simulink model "IB_BIEN_y_TG_BIEN"  (Simulink 8.1)
settings: Solver=ode45  StartTime=0.0  StopTime=50  RelTol=1e-3
PreLoadFcn:
  | Initial_datab
  | Const_IB
values from neighbouring files (symbols this model uses):
  a1 = (Iyy-Izz)/Ixx    (= -1.125)    [Initial_datab.m]
  a2 = Jr/Ixx    (= 0.00697115384615)    [Initial_datab.m]
  a3 = (Izz-Ixx)/Iyy    (= 1.11607142857)    [Initial_datab.m]
  a5 = (Ixx-Iyy)/Izz    (= -0.0349344978166)    [Initial_datab.m]
  alp1 = 20    [Initial_datab.m]
  alp2 = 10    [Initial_datab.m]
  b = 1.2*10^(-4)    (= 0.00012)    [Initial_datab.m]
  b1 = 1/Ixx    (= 96.1538461538)    [Initial_datab.m]
  b2 = 1/Iyy    (= 89.2857142857)    [Initial_datab.m]
  b3 = 1/Izz    (= 43.6681222707)    [Initial_datab.m]
  c1 = 10    [Const_IB.m]
  c10 = 0.75    [Const_IB.m]
  c11 = 1    [Const_IB.m]
  c12 = 0.75    [Const_IB.m]
  c2 = 6    [Const_IB.m]
  c3 = 10    [Const_IB.m]
  c4 = 6    [Const_IB.m]
  c5 = 2    [Const_IB.m]
  c6 = 2    [Const_IB.m]
  c7 = 3.5    [Const_IB.m]
  c8 = 1.5    [Const_IB.m]
  c9 = 1    [Const_IB.m]
  d = 3*10^(-6)    (= 3e-06)    [Initial_datab.m]
  Ixx = 10.4*10^(-3)    (= 0.0104)    [Initial_datab.m]
  Iyy = 11.2*10^(-3)    (= 0.0112)    [Initial_datab.m]
  Izz = 2.29*10^(-2)    (= 0.0229)    [Initial_datab.m]
  Jr = 7.25*10^(-5)    (= 7.25e-05)    [Initial_datab.m]
  k1x = -k1x    (= -0.5)    [Initial_datab.m]
  k1y = -k1y    (= -0.5)    [Initial_datab.m]
  k1z = -k1z    (= -2)    [Initial_datab.m]
  l = 0.225    [Initial_datab.m]
  ld1 = 0.07    [Const_IB.m]
  ld2 = 0.05    [Const_IB.m]
  ld3 = 0.01    [Const_IB.m]
  ld4 = 0.01    [Const_IB.m]
  ld5 = 0.001    [Const_IB.m]
  ld6 = 0.001    [Const_IB.m]
  m = 1.14    [Initial_datab.m]
  phi0 = 0    [Initial_datab.m]
  phi0dot = 0    [Initial_datab.m]
  psi0 = 0    [Initial_datab.m]
  psi0dot = 0    [Initial_datab.m]
  theta0 = 0    [Initial_datab.m]
  theta0dot = 0    [Initial_datab.m]
  x0 = 0    [Initial_datab.m]
  x0dot = 0    [Initial_datab.m]
  xf = -5    [Initial_datab.m]
  xfdot = 0    [Initial_datab.m]
  y0 = 0    [Initial_datab.m]
  y0dot = 0    [Initial_datab.m]
  yf = 5    [Initial_datab.m]
  yfdot = 0    [Initial_datab.m]
  z0 = 0    [Initial_datab.m]
  z0dot = 0    [Initial_datab.m]
  zf = 50    [Initial_datab.m]
  zfdot = 0    [Initial_datab.m]
undefined symbols (not defined in the file or in its folder): sigbuilder_block
(part 1 of 2)
settings Model: Creator=Ana  LastModifiedBy=Admin
settings SolverCC: MaxConsecutiveMinStep=5
settings DebuggingCC: StrictBusMsg=Warning

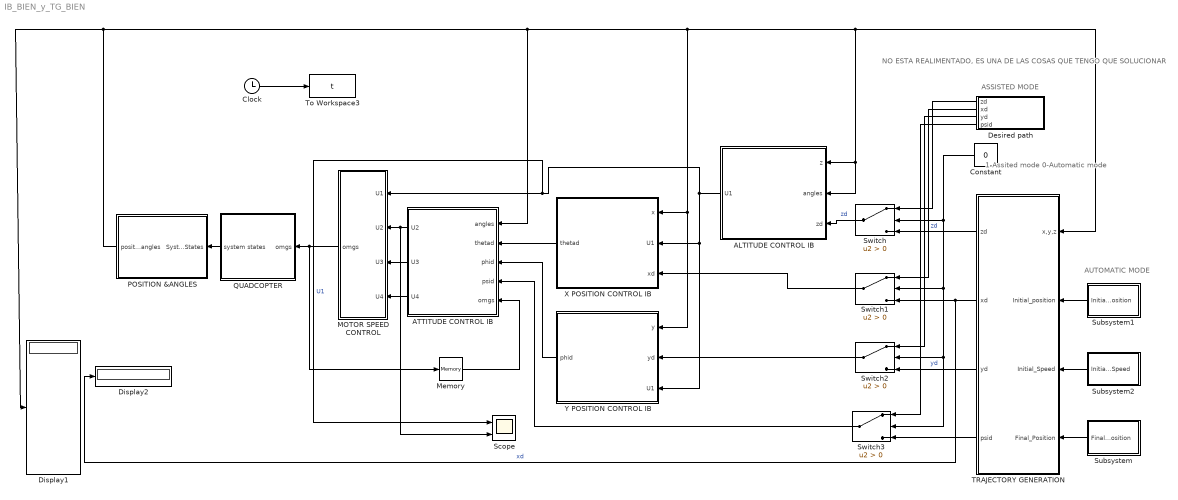
== system IB_BIEN_y_TG_BIEN ==
  note: ASSISTED MODE
  note: AUTOMATIC MODE
  note: 1-Assited mode
      | 0-Automatic mode
  note: NO ESTA REALIMENTADO,
      | ES UNA DE LAS COSAS QUE TENGO QUE SOLUCIONAR
  ALTITUDE CONTROL IB : Subsystem
  ATTITUDE CONTROL IB : Subsystem  TreatAsAtomicUnit=on
  Clock : Clock
  Constant : Constant  Value=0
  Desired path : Subsystem  Tag=STV Subsys  LoadFcn=sigbuilder_block('load');  StartFcn=sigbuilder_block('start');  StopFcn=sigbuilder_block('stop');  ClipboardFcn=sigbuilder_block('clipboard');  mask(Sigbuilder block){}
      mask help: Simulink:masks:SigbuilderBlock_MD
      mask init:
      | if ~strcmp(get_param(bdroot(gcbh),'SimulationStatus'),'stopped') tuvar = sigbuilder_block('maskInit'); end
      settings: CopyFcn=sigbuilder_block('copy');  DeleteFcn=sigbuilder_block('delete');  ModelCloseFcn=sigbuilder_block('modelClose');  PreSaveFcn=sigbuilder_block('preSave');  PauseFcn=sigbuilder_block('pause')  ContinueFcn=sigbuilder_block('continue')  NameChangeFcn=sigbuilder_block('namechange');  OpenFcn=sigbuilder_block('open',[6 28.5 1012.5 483.75 ]);  CloseFcn=sigbuilder_block('close');
      mask Display: plot(0, 0, 100, 100,[2, 2, 32, 32, 2], [68, 8, 8, 68, 68],[32, 2], [38, 38], [32, 19, 2],[53, 60, 44], [32, 17, 17, 2],[16, 16, 31, 31]);txt = getActiveGroup(gcbh);text(2, 100, txt,'verticalAlignment', 'top');
  Display1 : Display
  Display2 : Display
  MOTOR SPEED CONTROL : Subsystem
  Memory : Memory
  POSITION &ANGLES : Subsystem
  QUADCOPTER : Subsystem
  Scope : Scope  NumInputPorts=2
      settings: YMin=8~0  YMax=23~24  SaveName=ScopeData12
  Subsystem : Subsystem
  Subsystem1 : Subsystem
  Subsystem2 : Subsystem
  Switch{,1..3} (4 alike) : Switch  Criteria=u2 > Threshold
  TRAJECTORY GENERATION : Subsystem
  To Workspace3 : ToWorkspace  VariableName=t  SampleTime=-1
  X POSITION CONTROL IB : Subsystem  TreatAsAtomicUnit=on
  Y POSITION CONTROL IB : Subsystem  TreatAsAtomicUnit=on
  wires:
  QUADCOPTER/1(system states) -> POSITION &ANGLES/1(SystemStates)
  ATTITUDE CONTROL IB/1(U2) -> Scope/2, MOTOR SPEED CONTROL/2(U2)
  MOTOR SPEED CONTROL/1(omgs) -> QUADCOPTER/1(omgs), Memory/1
  Y POSITION CONTROL IB/1(phid) -> ATTITUDE CONTROL IB/3(phid)
  Memory/1 -> ATTITUDE CONTROL IB/5(omgs)
  Clock/1 -> To Workspace3/1
  ALTITUDE CONTROL IB/1(U1) -> Scope/1, MOTOR SPEED CONTROL/1(U1), X POSITION CONTROL IB/2(U1), Y POSITION CONTROL IB/3(U1)  "U1"
  ATTITUDE CONTROL IB/2(U3) -> MOTOR SPEED CONTROL/3(U3)
  ATTITUDE CONTROL IB/3(U4) -> MOTOR SPEED CONTROL/4(U4)
  Subsystem/1(Final Position) -> TRAJECTORY GENERATION/4(Final_Position)
  Subsystem2/1(Initial Speed) -> TRAJECTORY GENERATION/3(Initial_Speed)
  Subsystem1/1(Initial Position) -> TRAJECTORY GENERATION/2(Initial_position)
  X POSITION CONTROL IB/1(thetad) -> ATTITUDE CONTROL IB/2(thetad)
  Switch/1 -> ALTITUDE CONTROL IB/3(zd)  "zd"
  TRAJECTORY GENERATION/1(zd) -> Switch/3  "zd"
  Desired path/1(zd) -> Switch/1
  Switch1/1 -> X POSITION CONTROL IB/3(xd)
  Switch2/1 -> Y POSITION CONTROL IB/2(yd)
  TRAJECTORY GENERATION/2(xd) -> Display2/1, Switch1/3  "xd"
  TRAJECTORY GENERATION/3(yd) -> Switch2/3  "yd"
  Desired path/2(xd) -> Switch1/1
  Desired path/3(yd) -> Switch2/1
  Constant/1 -> Switch/2, Switch1/2, Switch2/2, Switch3/2
  Switch3/1 -> ATTITUDE CONTROL IB/4(psid)
  Desired path/4(psid) -> Switch3/1
  TRAJECTORY GENERATION/4(psid) -> Switch3/3
  POSITION &ANGLES/1(position&angles) -> X POSITION CONTROL IB/1(x), Y POSITION CONTROL IB/1(y), ALTITUDE CONTROL IB/1(z), ALTITUDE CONTROL IB/2(angles), TRAJECTORY GENERATION/1(x,y,z), ATTITUDE CONTROL IB/1(angles), Display1/1

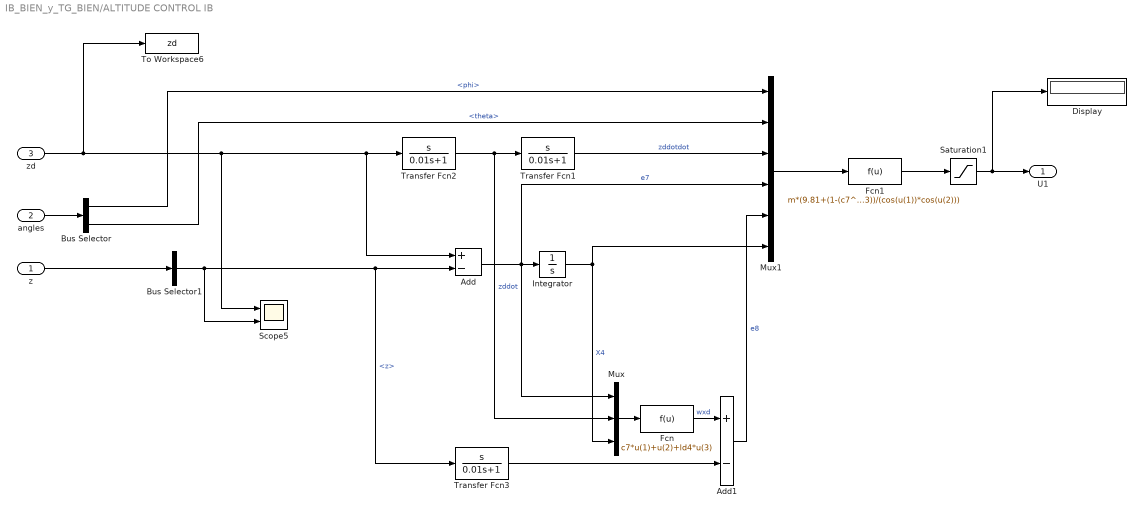
== system IB_BIEN_y_TG_BIEN/ALTITUDE CONTROL IB ==
  z : Inport
  angles : Inport  Port=2
  zd : Inport  Port=3
  Add : Sum  Inputs=+-
  Add1 : Sum  Inputs=+-
  Bus Selector : BusSelector  OutputSignals=phi,theta
  Bus Selector1 : BusSelector  OutputSignals=z
  Display : Display
  Fcn : Fcn  Expr=c7*u(1)+u(2)+ld4*u(3)
  Fcn1 : Fcn  Expr=m*(9.81+(1-(c7^2)+ld4)*u(4)+(c7+c8)*u(5)-c7*ld4*u(6)+u(3))/(cos(u(1))*cos(u(2)))
  Integrator : Integrator
  Mux : Mux  Inputs=3
  Mux1 : Mux  Inputs=6
  Saturation1 : Saturate  UpperLimit=22.36  LowerLimit=0
  Scope5 : Scope  NumInputPorts=2
      settings: YMin=-5~-5  YMax=5~5  SaveName=ScopeData11
  To Workspace6 : ToWorkspace  VariableName=zd  SampleTime=-1
  Transfer Fcn1 : TransferFcn  Numerator=[1 0]  Denominator=[0.01 1]
  Transfer Fcn2 : TransferFcn  Numerator=[1 0]  Denominator=[0.01 1]
  Transfer Fcn3 : TransferFcn  Numerator=[1 0]  Denominator=[0.01 1]
  U1 : Outport
  wires:
  zd/1 -> Scope5/1, Add/1, Transfer Fcn2/1, To Workspace6/1
  Transfer Fcn2/1 -> Mux/2, Transfer Fcn1/1  "zddot"
  Add/1 -> Integrator/1, Mux/1, Mux1/4  "e7"
  Integrator/1 -> Mux/3, Mux1/6  "X4"
  Fcn/1 -> Add1/1  "wxd"
  Mux/1 -> Fcn/1
  Mux1/1 -> Fcn1/1
  Fcn1/1 -> Saturation1/1
  Transfer Fcn3/1 -> Add1/2
  Transfer Fcn1/1 -> Mux1/3  "zddotdot"
  Add1/1 -> Mux1/5  "e8"
  angles/1 -> Bus Selector/1
  Bus Selector/1 -> Mux1/1  "<phi>"
  Bus Selector/2 -> Mux1/2  "<theta>"
  z/1 -> Bus Selector1/1
  Bus Selector1/1 -> Scope5/2, Add/2, Transfer Fcn3/1  "<z>"
  Saturation1/1 -> Display/1, U1/1

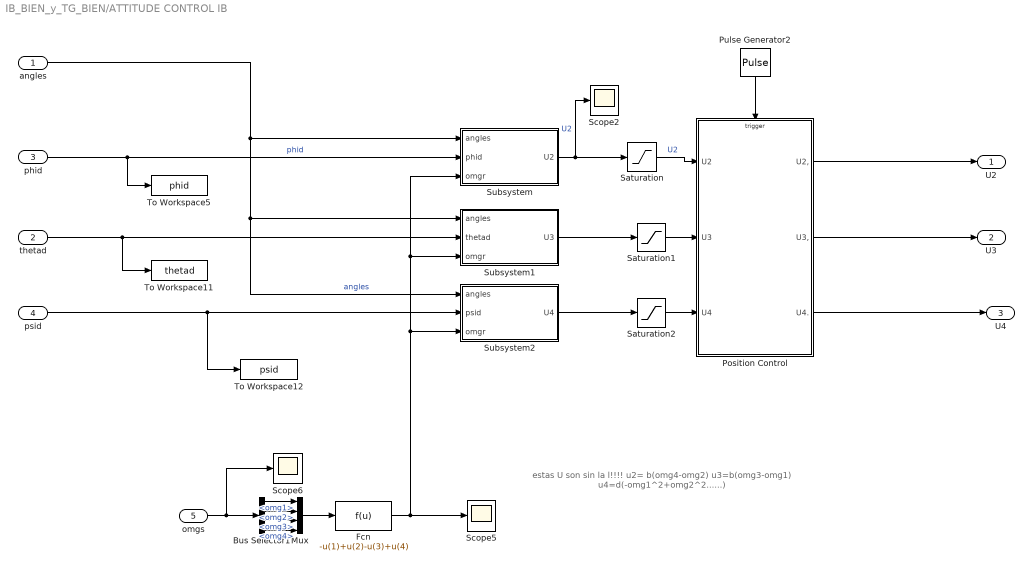
== system IB_BIEN_y_TG_BIEN/ATTITUDE CONTROL IB ==
  note: estas U son sin la l!!!!
      | u2= b(omg4-omg2)
      | u3=b(omg3-omg1)
      | u4=d(-omg1^2+omg2^2......)
  angles : Inport
  thetad : Inport  Port=2
  phid : Inport  Port=3
  psid : Inport  Port=4
  omgs : Inport  Port=5
  Bus Selector1 : BusSelector  OutputSignals=omg1,omg2,omg3,omg4
  Fcn : Fcn  Expr=-u(1)+u(2)-u(3)+u(4)
  Mux : Mux
  Position Control : Subsystem  TreatAsAtomicUnit=on
  Pulse Generator2 : DiscretePulseGenerator  PulseType=Time based  Period=0.0264  PulseWidth=50  SampleTime=[0.1, 0]
  Saturation : Saturate  UpperLimit=5.5915  LowerLimit=-5.5915
  Saturation1 : Saturate  UpperLimit=5.5915  LowerLimit=-5.5915
  Saturation2 : Saturate  UpperLimit=5.5915  LowerLimit=-5.5915
  Scope2 : Scope
      settings: SaveName=ScopeData40
  Scope5 : Scope
      settings: SaveName=ScopeData43
  Scope6 : Scope
      settings: TimeRange=1.202697773920718e-023  YMin=0  YMax=250  SaveName=ScopeData44
  Subsystem : Subsystem
  Subsystem1 : Subsystem
  Subsystem2 : Subsystem
  To Workspace11 : ToWorkspace  VariableName=thetad  SampleTime=-1
  To Workspace12 : ToWorkspace  VariableName=psid  SampleTime=-1
  To Workspace5 : ToWorkspace  VariableName=phid  SampleTime=-1
  U2 : Outport
  U3 : Outport  Port=2
  U4 : Outport  Port=3
  wires:
  phid/1 -> Subsystem/2(phid), To Workspace5/1  "phid"
  Position Control/1(U2,) -> U2/1
  Subsystem/1(U2) -> Scope2/1, Saturation/1  "U2"
  omgs/1 -> Bus Selector1/1, Scope6/1
  Bus Selector1/1 -> Mux/1  "<omg1>"
  Bus Selector1/2 -> Mux/2  "<omg2>"
  Bus Selector1/3 -> Mux/3  "<omg3>"
  Bus Selector1/4 -> Mux/4  "<omg4>"
  Mux/1 -> Fcn/1
  Fcn/1 -> Scope5/1, Subsystem/3(omgr), Subsystem1/3(omgr), Subsystem2/3(omgr)
  Pulse Generator2/1 -> Position Control/Trigger
  Saturation/1 -> Position Control/1(U2)  "U2"
  thetad/1 -> Subsystem1/2(thetad), To Workspace11/1
  Subsystem1/1(U3) -> Saturation1/1
  Position Control/2(U3,) -> U3/1
  angles/1 -> Subsystem/1(angles), Subsystem1/1(angles), Subsystem2/1(angles)  "angles"
  Saturation1/1 -> Position Control/2(U3)
  Subsystem2/1(U4) -> Saturation2/1
  Saturation2/1 -> Position Control/3(U4)
  Position Control/3(U4.) -> U4/1
  psid/1 -> Subsystem2/2(psid), To Workspace12/1

== system IB_BIEN_y_TG_BIEN/Desired path ==
  Demux : Demux  Tag=STV Demux
  FromWs : FromWorkspace  Tag=STV FromWs  VariableName=tuvar  SampleTime=0  SigBuilderData=DataTag0  VnvData=DataTag1
      SigBuilderData=|
      | common.afterFinalStr = 'Extrapolate'
      | common.sampleTime = 0
      | dataSet.timeRange = [0 30]
      | dataSet.name = 'Group 1'
      | sbobj.Groups.Name = 'Group 1'
      | sbobj.Groups.Signals(1).Name = 'zd'
      | sbobj.Groups.Signals(1).XData = [0 5 20 20 30]
      | sbobj.Groups.Signals(1).YData = [0 0 1 2 2]
      | sbobj.Groups.Signals(2).Name = 'xd'
      | sbobj.Groups.Signals(2).XData = [0 5 5 30]
      | sbobj.Groups.Signals(2).YData = [0 0 1 1]
      | sbobj.Groups.Signals(3).Name = 'yd'
      | sbobj.Groups.Signals(3).XData = [0 5 10 18 18 30]
      | sbobj.Groups.Signals(3).YData = [0 0.02 0.1 0.3 0.5 0]
      | sbobj.Groups.Signals(4).Name = 'psid'
      | sbobj.Groups.Signals(4).XData = [0 12 18 25 30]
      | sbobj.Groups.Signals(4).YData = [0 0.5 0.5 0.5 0.5]
      | sbobj.Groups.TimeRange = [0 30]
  zd : Outport  Tag=STV Outport
  xd : Outport  Tag=STV Outport  Port=2
  yd : Outport  Tag=STV Outport  Port=3
  psid : Outport  Tag=STV Outport  Port=4
  wires:
  FromWs/1 -> Demux/1
  Demux/1 -> zd/1
  Demux/2 -> xd/1
  Demux/3 -> yd/1
  Demux/4 -> psid/1

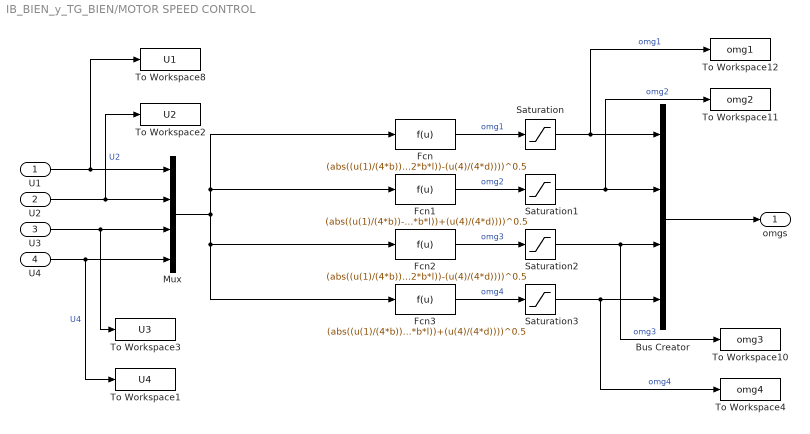
== system IB_BIEN_y_TG_BIEN/MOTOR SPEED CONTROL ==
  U1 : Inport
  U2 : Inport  Port=2
  U3 : Inport  Port=3
  U4 : Inport  Port=4
  Bus Creator : BusCreator
  Fcn : Fcn  Expr=(abs((u(1)/(4*b))-(u(3)/(2*b*l))-(u(4)/(4*d))))^0.5
  Fcn1 : Fcn  Expr=(abs((u(1)/(4*b))-(u(2)/(2*b*l))+(u(4)/(4*d))))^0.5
  Fcn2 : Fcn  Expr=(abs((u(1)/(4*b))+(u(3)/(2*b*l))-(u(4)/(4*d))))^0.5
  Fcn3 : Fcn  Expr=(abs((u(1)/(4*b))+(u(2)/(2*b*l))+(u(4)/(4*d))))^0.5
  Mux : Mux
  Saturation{,1..3} (4 alike) : Saturate  UpperLimit=215.86  LowerLimit=0
  To Workspace1 : ToWorkspace  VariableName=U4  SampleTime=-1
  To Workspace10 : ToWorkspace  VariableName=omg3  SampleTime=-1
  To Workspace11 : ToWorkspace  VariableName=omg2  SampleTime=-1
  To Workspace12 : ToWorkspace  VariableName=omg1  SampleTime=-1
  To Workspace2 : ToWorkspace  VariableName=U2  SampleTime=-1
  To Workspace3 : ToWorkspace  VariableName=U3  SampleTime=-1
  To Workspace4 : ToWorkspace  VariableName=omg4  SampleTime=-1
  To Workspace8 : ToWorkspace  VariableName=U1  SampleTime=-1
  omgs : Outport
  wires:
  U2/1 -> Mux/2, To Workspace2/1  "U2"
  Bus Creator/1 -> omgs/1
  U1/1 -> Mux/1, To Workspace8/1
  Mux/1 -> Fcn3/1, Fcn2/1, Fcn/1, Fcn1/1
  Fcn/1 -> Saturation/1  "omg1"
  Fcn1/1 -> Saturation1/1  "omg2"
  Fcn2/1 -> Saturation2/1  "omg3"
  Fcn3/1 -> Saturation3/1  "omg4"
  Saturation/1 -> Bus Creator/1, To Workspace12/1  "omg1"
  Saturation1/1 -> Bus Creator/2, To Workspace11/1  "omg2"
  Saturation2/1 -> Bus Creator/3, To Workspace10/1  "omg3"
  Saturation3/1 -> Bus Creator/4, To Workspace4/1  "omg4"
  U3/1 -> Mux/3, To Workspace3/1
  U4/1 -> Mux/4, To Workspace1/1  "U4"

== system IB_BIEN_y_TG_BIEN/POSITION &ANGLES ==
  SystemStates : Inport
  Bus Creator : BusCreator  Inputs=9
  Bus Selector : BusSelector  OutputSignals=x,y,z,phi,theta,psi,phidot,thetadot,psidot
  To Workspace10 : ToWorkspace  VariableName=theta  SampleTime=-1
  To Workspace13 : ToWorkspace  VariableName=psi  SampleTime=-1
  To Workspace2 : ToWorkspace  VariableName=y  SampleTime=-1
  To Workspace4 : ToWorkspace  VariableName=phi  SampleTime=-1
  To Workspace7 : ToWorkspace  VariableName=z  SampleTime=-1
  To Workspace9 : ToWorkspace  VariableName=x  SampleTime=-1
  position&angles : Outport
  wires:
  SystemStates/1 -> Bus Selector/1
  Bus Creator/1 -> position&angles/1  "position&angles"
  Bus Selector/1 -> Bus Creator/1, To Workspace9/1  "<x>"
  Bus Selector/2 -> Bus Creator/2, To Workspace2/1  "<y>"
  Bus Selector/3 -> Bus Creator/3, To Workspace7/1  "<z>"
  Bus Selector/4 -> Bus Creator/4, To Workspace4/1  "<phi>"
  Bus Selector/5 -> Bus Creator/5, To Workspace10/1  "<theta>"
  Bus Selector/6 -> Bus Creator/6, To Workspace13/1  "<psi>"
  Bus Selector/7 -> Bus Creator/7  "<phidot>"
  Bus Selector/8 -> Bus Creator/8  "<thetadot>"
  Bus Selector/9 -> Bus Creator/9  "<psidot>"

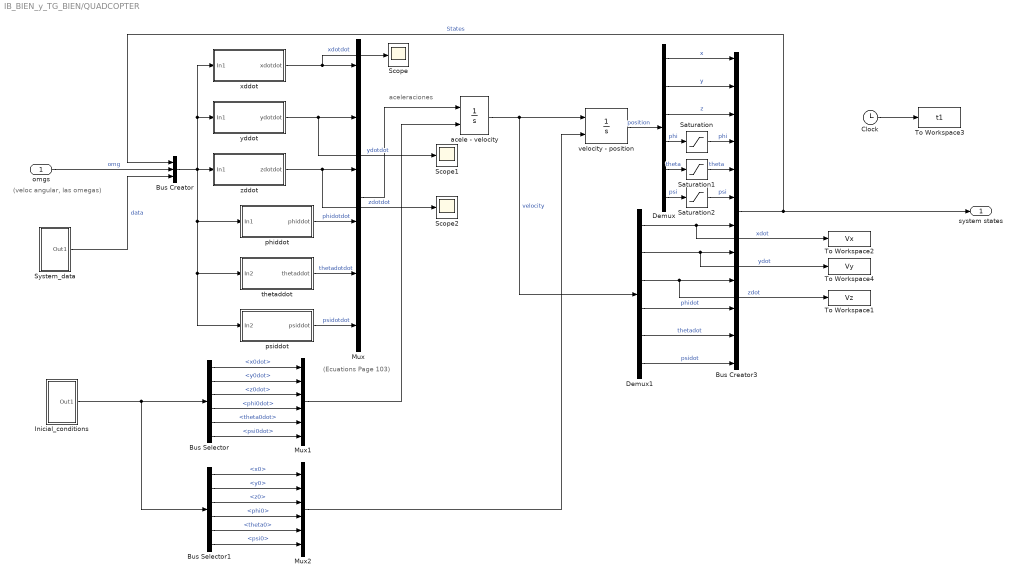
== system IB_BIEN_y_TG_BIEN/QUADCOPTER ==
  note: aceleraciones
  note: (Ecuations Page 103)
  note: (veloc angular, las omegas)
  omgs : Inport
  Bus Creator : BusCreator  Inputs=3
  Bus Creator3 : BusCreator  Inputs=12
  Bus Selector : BusSelector  OutputSignals=x0dot,y0dot,z0dot,phi0dot,theta0dot,psi0dot
  Bus Selector1 : BusSelector  OutputSignals=x0,y0,z0,phi0,theta0,psi0
  Clock : Clock
  Demux : Demux  Outputs=6
  Demux1 : Demux  Outputs=6
  Inicial_conditions : Subsystem
  Mux : Mux  Inputs=6
  Mux1 : Mux  Inputs=6
  Mux2 : Mux  Inputs=6
  Saturation : Saturate  UpperLimit=0.7854  LowerLimit=-0.7854
  Saturation1 : Saturate  UpperLimit=0.7854  LowerLimit=-0.7854
  Saturation2 : Saturate  UpperLimit=0.7854  LowerLimit=-0.7854
  Scope : Scope
      settings: SaveName=ScopeData7
  Scope1 : Scope
      settings: SaveName=ScopeData8
  Scope2 : Scope
      settings: SaveName=ScopeData9
  System_data : Subsystem
  To Workspace1 : ToWorkspace  VariableName=Vz  SampleTime=-1
  To Workspace2 : ToWorkspace  VariableName=Vx  SampleTime=-1
  To Workspace3 : ToWorkspace  VariableName=t1  SampleTime=-1
  To Workspace4 : ToWorkspace  VariableName=Vy  SampleTime=-1
  acele - velocity : Integrator  InitialConditionSource=external  UpperSaturationLimit=Inf  LowerSaturationLimit=-Inf
  phiddot : Subsystem
  psiddot : Subsystem
  thetaddot : Subsystem
  velocity - position : Integrator  InitialConditionSource=external
  xddot : Subsystem
  yddot : Subsystem
  zddot : Subsystem
  system states : Outport
  wires:
  Bus Creator3/1 -> Bus Creator/1, system states/1  "States"
  Mux1/1 -> acele - velocity/2
  velocity - position/1 -> Demux/1  "position"
  Mux2/1 -> velocity - position/2
  acele - velocity/1 -> velocity - position/1, Demux1/1  "velocity"
  Mux/1 -> acele - velocity/1
  omgs/1 -> Bus Creator/2  "omg"
  System_data/1(Out1) -> Bus Creator/3  "data"
  Bus Creator/1 -> phiddot/1(In1), thetaddot/1(In2), psiddot/1(In2), yddot/1(In1), xddot/1(In1), zddot/1(In1)
  Inicial_conditions/1(Out1) -> Bus Selector/1, Bus Selector1/1
  Clock/1 -> To Workspace3/1
  Bus Selector/1 -> Mux1/1  "<x0dot>"
  Bus Selector/2 -> Mux1/2  "<y0dot>"
  Bus Selector/3 -> Mux1/3  "<z0dot>"
  Bus Selector/4 -> Mux1/4  "<phi0dot>"
  Bus Selector/5 -> Mux1/5  "<theta0dot>"
  Bus Selector1/1 -> Mux2/1  "<x0>"
  Bus Selector1/2 -> Mux2/2  "<y0>"
  Bus Selector1/3 -> Mux2/3  "<z0>"
  Bus Selector1/4 -> Mux2/4  "<phi0>"
  Bus Selector1/5 -> Mux2/5  "<theta0>"
  xddot/1(xdotdot) -> Mux/1, Scope/1  "xdotdot"
  yddot/1(ydotdot) -> Mux/2, Scope1/1  "ydotdot"
  zddot/1(zdotdot) -> Mux/3, Scope2/1  "zdotdot"
  phiddot/1(phiddot) -> Mux/4  "phidotdot"
  thetaddot/1(thetaddot) -> Mux/5  "thetadotdot"
  Demux/2 -> Bus Creator3/2  "y"
  Demux/3 -> Bus Creator3/3  "z"
  Demux/4 -> Saturation/1  "phi"
  Demux/5 -> Saturation1/1  "theta"
  Demux/1 -> Bus Creator3/1  "x"
  Saturation/1 -> Bus Creator3/4  "phi"
  Saturation1/1 -> Bus Creator3/5  "theta"
  Bus Selector/6 -> Mux1/6  "<psi0dot>"
  Bus Selector1/6 -> Mux2/6  "<psi0>"
  psiddot/1(psiddot) -> Mux/6  "psidotdot"
  Demux/6 -> Saturation2/1  "psi"
  Saturation2/1 -> Bus Creator3/6  "psi"
  Demux1/1 -> Bus Creator3/7, To Workspace2/1  "xdot"
  Demux1/2 -> Bus Creator3/8, To Workspace4/1  "ydot"
  Demux1/3 -> Bus Creator3/9, To Workspace1/1  "zdot"
  Demux1/4 -> Bus Creator3/10  "phidot"
  Demux1/5 -> Bus Creator3/11  "thetadot"
  Demux1/6 -> Bus Creator3/12  "psidot"

== system IB_BIEN_y_TG_BIEN/Subsystem ==
  Bus Creator : BusCreator  Inputs=6
  Constant : Constant  Value=xf
  Constant1 : Constant  Value=yf
  Constant2 : Constant  Value=zf
  Constant3 : Constant  Value=xfdot
  Constant4 : Constant  Value=yfdot
  Constant5 : Constant  Value=zfdot
  Final Position : Outport
  wires:
  Bus Creator/1 -> Final Position/1
  Constant1/1 -> Bus Creator/2  "yf"
  Constant2/1 -> Bus Creator/3  "zf"
  Constant/1 -> Bus Creator/1  "xf"
  Constant3/1 -> Bus Creator/4  "xfdot"
  Constant4/1 -> Bus Creator/5  "yfdot"
  Constant5/1 -> Bus Creator/6  "zfdot"

== system IB_BIEN_y_TG_BIEN/Subsystem1 ==
  Bus Creator : BusCreator  Inputs=3
  Constant : Constant  Value=x0
  Constant1 : Constant  Value=y0
  Constant2 : Constant  Value=z0
  Initial Position : Outport
  wires:
  Constant1/1 -> Bus Creator/2  "y0"
  Constant/1 -> Bus Creator/1  "x0"
  Bus Creator/1 -> Initial Position/1
  Constant2/1 -> Bus Creator/3  "z0"

== system IB_BIEN_y_TG_BIEN/Subsystem2 ==
  Bus Creator : BusCreator  Inputs=3
  Constant3 : Constant  Value=x0dot
  Constant4 : Constant  Value=y0dot
  Constant5 : Constant  Value=z0dot
  Initial Speed : Outport
  wires:
  Bus Creator/1 -> Initial Speed/1
  Constant5/1 -> Bus Creator/3  "z0dot"
  Constant3/1 -> Bus Creator/1  "x0dot"
  Constant4/1 -> Bus Creator/2  "y0dot"

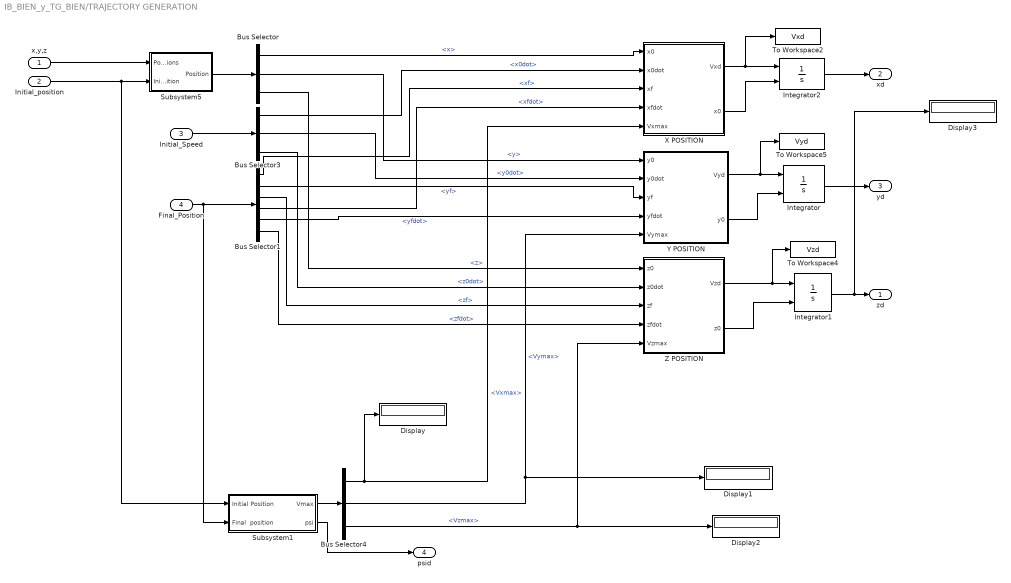
== system IB_BIEN_y_TG_BIEN/TRAJECTORY GENERATION ==
  x,y,z : Inport
  Initial_position : Inport  Port=2
  Initial_Speed : Inport  Port=3
  Final_Position : Inport  Port=4
  Bus Selector : BusSelector  OutputSignals=x,y,z
  Bus Selector1 : BusSelector  OutputSignals=xf,yf,zf,xfdot,yfdot,zfdot
  Bus Selector3 : BusSelector  OutputSignals=x0dot,y0dot,z0dot
  Bus Selector4 : BusSelector  OutputSignals=Vxmax,Vymax,Vzmax
  Display{,1..3} (4 alike) : Display
  Integrator : Integrator  InitialConditionSource=external
  Integrator1 : Integrator  InitialConditionSource=external
  Integrator2 : Integrator  InitialConditionSource=external
  Subsystem1 : Subsystem
  Subsystem5 : Subsystem
  To Workspace2 : ToWorkspace  VariableName=Vxd  SampleTime=-1
  To Workspace4 : ToWorkspace  VariableName=Vzd  SampleTime=-1
  To Workspace5 : ToWorkspace  VariableName=Vyd  SampleTime=-1
  X POSITION : Subsystem
  Y POSITION : Subsystem
  Z POSITION : Subsystem
  zd : Outport
  xd : Outport  Port=2
  yd : Outport  Port=3
  psid : Outport  Port=4
  wires:
  Bus Selector/1 -> X POSITION/1(x0)  "<x>"
  Bus Selector1/1 -> X POSITION/3(xf)  "<xf>"
  Bus Selector3/1 -> X POSITION/2(x0dot)  "<x0dot>"
  Bus Selector1/4 -> X POSITION/4(xfdot)  "<xfdot>"
  Bus Selector/2 -> Y POSITION/1(y0)  "<y>"
  Bus Selector3/2 -> Y POSITION/2(y0dot)  "<y0dot>"
  Bus Selector1/2 -> Y POSITION/3(yf)  "<yf>"
  Bus Selector1/5 -> Y POSITION/4(yfdot)  "<yfdot>"
  Bus Selector/3 -> Z POSITION/1(z0)  "<z>"
  Bus Selector3/3 -> Z POSITION/2(z0dot)  "<z0dot>"
  Bus Selector1/3 -> Z POSITION/3(zf)  "<zf>"
  Bus Selector1/6 -> Z POSITION/4(zfdot)  "<zfdot>"
  X POSITION/1(Vxd) -> To Workspace2/1, Integrator2/1
  Subsystem5/1(Position) -> Bus Selector/1
  Final_Position/1 -> Bus Selector1/1, Subsystem1/2(Final  position)
  Z POSITION/1(Vzd) -> To Workspace4/1, Integrator1/1
  Initial_Speed/1 -> Bus Selector3/1
  Y POSITION/1(Vyd) -> To Workspace5/1, Integrator/1
  Initial_position/1 -> Subsystem5/2(Initial_position), Subsystem1/1(Initial Position)
  x,y,z/1 -> Subsystem5/1(Positions)
  Subsystem1/1(Vmax) -> Bus Selector4/1
  Bus Selector4/1 -> Display/1, X POSITION/5(Vxmax)  "<Vxmax>"
  Bus Selector4/2 -> Display1/1, Y POSITION/5(Vymax)  "<Vymax>"
  Bus Selector4/3 -> Display2/1, Z POSITION/5(Vzmax)  "<Vzmax>"
  Integrator2/1 -> xd/1
  Integrator/1 -> yd/1
  Integrator1/1 -> Display3/1, zd/1
  X POSITION/2("x0 ") -> Integrator2/2
  Y POSITION/2("y0  ") -> Integrator/2
  Z POSITION/2("z0 ") -> Integrator1/2
  Subsystem1/2(psi) -> psid/1

== system IB_BIEN_y_TG_BIEN/X POSITION CONTROL IB ==
  x : Inport
  U1 : Inport  Port=2
  xd : Inport  Port=3
  Bus Selector : BusSelector  OutputSignals=x
  Position Control : Subsystem  TreatAsAtomicUnit=on
  Pulse Generator1 : DiscretePulseGenerator  PulseType=Time based  Period=0.04  PulseWidth=50
  Saturation2 : Saturate  UpperLimit=0.7854  LowerLimit=-0.7854
  Subsystem1 : Subsystem
  To Workspace8 : ToWorkspace  VariableName=xd  SampleTime=-1
  thetad : Outport
  wires:
  U1/1 -> Subsystem1/3(U1)
  Subsystem1/1(thetad) -> Position Control/1(In2)  "thetad"
  Pulse Generator1/1 -> Position Control/Trigger
  Position Control/1(thetad) -> Saturation2/1
  xd/1 -> Subsystem1/2(xd), To Workspace8/1  "xd"
  x/1 -> Bus Selector/1  "x"
  Bus Selector/1 -> Subsystem1/1(x)  "<x>"
  Saturation2/1 -> thetad/1

== system IB_BIEN_y_TG_BIEN/Y POSITION CONTROL IB ==
  y : Inport
  yd : Inport  Port=2
  U1 : Inport  Port=3
  Bus Selector : BusSelector  OutputSignals=y
  Position Control : Subsystem  TreatAsAtomicUnit=on
  Pulse Generator1 : DiscretePulseGenerator  PulseType=Time based  Period=0.04  PulseWidth=50
  Saturation : Saturate  UpperLimit=0.7854  LowerLimit=-0.7854
  Scope : Scope
  Subsystem1 : Subsystem
  To Workspace1 : ToWorkspace  VariableName=yd  SampleTime=-1
  phid : Outport
  wires:
  U1/1 -> Subsystem1/3(U1), Scope/1
  Subsystem1/1(phid) -> Position Control/1(In2)  "phid"
  Pulse Generator1/1 -> Position Control/Trigger
  Position Control/1(phid) -> Saturation/1
  yd/1 -> Subsystem1/2(yd), To Workspace1/1  "yd"
  y/1 -> Bus Selector/1
  Bus Selector/1 -> Subsystem1/1(y)  "<y>"
  Saturation/1 -> phid/1

== system IB_BIEN_y_TG_BIEN/ATTITUDE CONTROL IB/Position Control ==
  U2 : Inport
  U3 : Inport  Port=2
  U4 : Inport  Port=3
  Trigger : TriggerPort  PortDimensions=1
  U2, : Outport
  U3, : Outport  Port=2
  U4. : Outport  Port=3
  wires:
  U2/1 -> U2,/1
  U3/1 -> U3,/1
  U4/1 -> U4./1

== system IB_BIEN_y_TG_BIEN/ATTITUDE CONTROL IB/Subsystem ==
  angles : Inport
  phid : Inport  Port=2
  omgr : Inport  Port=3
  Add : Sum  Inputs=+-
  Add1 : Sum  Inputs=+-
  Bus Selector : BusSelector  OutputSignals=phi,thetadot,psidot
  Fcn : Fcn  Expr=c1*u(1)+u(2)+ld1*u(3)
  Fcn1 : Fcn  Expr=((1-(c1^2)+ld1)*u(5)+(c1+c2)*u(6)-c1*ld1*u(4)+u(3)-(u(1)*u(2)*a1)+(u(1)*a2*u(7)))/b1
  Integrator : Integrator
  Mux : Mux  Inputs=3
  Mux1 : Mux  Inputs=7
  Scope{1..2,4,6} (4 alike) : Scope
      Scope1 settings: TimeRange=1.202697773920718e-023  YMin=0  YMax=250  SaveName=ScopeData22
      Scope2 settings: TimeRange=1.202697773920718e-023  YMin=0  YMax=250  SaveName=ScopeData28
      Scope4 settings: TimeRange=1.202697773920718e-023  YMin=0  YMax=250  SaveName=ScopeData30
      Scope6 settings: TimeRange=1.202697773920718e-023  YMin=0  YMax=250  SaveName=ScopeData21
  Transfer Fcn2 : TransferFcn  Numerator=[1 0]  Denominator=[0.05 1]
  Transfer Fcn3 : TransferFcn  Numerator=[1 0]  Denominator=[0.01 1]
  Transfer Fcn4 : TransferFcn  Numerator=[1 0]  Denominator=[0.01 1]
  U2 : Outport
  wires:
  angles/1 -> Bus Selector/1
  phid/1 -> Add/1, Transfer Fcn2/1
  Transfer Fcn2/1 -> Mux/2, Transfer Fcn3/1  "phiddot"
  Bus Selector/1 -> Add/2, Transfer Fcn4/1  "<phi>"
  Add/1 -> Mux/1, Integrator/1, Mux1/5, Scope6/1  "e1"
  Integrator/1 -> Mux/3, Mux1/4, Scope1/1  "X1"
  Add1/1 -> Mux1/6, Scope2/1  "e2"
  Fcn/1 -> Add1/1  "wxd"
  Mux/1 -> Fcn/1
  Mux1/1 -> Fcn1/1
  Transfer Fcn3/1 -> Mux1/3  "phiddotdot"
  Fcn1/1 -> U2/1, Scope4/1
  Transfer Fcn4/1 -> Add1/2
  omgr/1 -> Mux1/7
  Bus Selector/2 -> Mux1/1  "<thetadot>"
  Bus Selector/3 -> Mux1/2  "<psidot>"

== system IB_BIEN_y_TG_BIEN/ATTITUDE CONTROL IB/Subsystem1 ==
  angles : Inport
  thetad : Inport  Port=2
  omgr : Inport  Port=3
  Add : Sum  Inputs=+-
  Add1 : Sum  Inputs=+-
  Bus Selector : BusSelector  OutputSignals=theta,phidot,psidot
  Fcn : Fcn  Expr=c1*u(1)+u(2)+ld1*u(3)
  Fcn1 : Fcn  Expr=((1-(c3^2)+ld2)*u(5)+(c3+c4)*u(6)-c3*ld2*u(4)+u(3)-(u(1)*u(2)*a3)-(u(1)*a2*u(7)))/b2
  Integrator : Integrator
  Mux : Mux  Inputs=3
  Mux1 : Mux  Inputs=7
  Scope{1..2,4,6} (4 alike) : Scope
      Scope1 settings: TimeRange=1.202697773920718e-023  YMin=0  YMax=250  SaveName=ScopeData22
      Scope2 settings: TimeRange=1.202697773920718e-023  YMin=0  YMax=250  SaveName=ScopeData28
      Scope4 settings: TimeRange=1.202697773920718e-023  YMin=0  YMax=250  SaveName=ScopeData30
      Scope6 settings: TimeRange=1.202697773920718e-023  YMin=0  YMax=250  SaveName=ScopeData21
  Transfer Fcn2 : TransferFcn  Numerator=[1 0]  Denominator=[0.05 1]
  Transfer Fcn3 : TransferFcn  Numerator=[1 0]  Denominator=[0.01 1]
  Transfer Fcn4 : TransferFcn  Numerator=[1 0]  Denominator=[0.01 1]
  U3 : Outport
  wires:
  angles/1 -> Bus Selector/1
  thetad/1 -> Add/1, Transfer Fcn2/1
  Transfer Fcn2/1 -> Mux/2, Transfer Fcn3/1  "thetaddot"
  Bus Selector/1 -> Add/2, Transfer Fcn4/1  "<theta>"
  Add/1 -> Mux/1, Integrator/1, Mux1/5, Scope6/1  "e3"
  Integrator/1 -> Mux/3, Mux1/4, Scope1/1  "X2"
  Add1/1 -> Mux1/6, Scope2/1  "e4"
  Fcn/1 -> Add1/1  "wxd"
  Mux/1 -> Fcn/1
  Mux1/1 -> Fcn1/1
  Transfer Fcn3/1 -> Mux1/3  "thetaddotdot"
  Fcn1/1 -> U3/1, Scope4/1
  Transfer Fcn4/1 -> Add1/2
  omgr/1 -> Mux1/7
  Bus Selector/2 -> Mux1/1  "<phidot>"
  Bus Selector/3 -> Mux1/2  "<psidot>"

== system IB_BIEN_y_TG_BIEN/ATTITUDE CONTROL IB/Subsystem2 ==
  angles : Inport
  psid : Inport  Port=2
  omgr : Inport  Port=3
  Add : Sum  Inputs=+-
  Add1 : Sum  Inputs=+-
  Bus Selector : BusSelector  OutputSignals=psi,phidot,thetadot
  Fcn : Fcn  Expr=c1*u(1)+u(2)+ld1*u(3)
  Fcn1 : Fcn  Expr=((1-(c5^2)+ld3)*u(5)+(c5+c6)*u(6)-c5*ld3*u(4)+u(3)-(u(1)*u(2)*a5))/b3
  Integrator : Integrator
  Mux : Mux  Inputs=3
  Mux1 : Mux  Inputs=7
  Scope{1..2,4,6} (4 alike) : Scope
      Scope1 settings: TimeRange=1.202697773920718e-023  YMin=0  YMax=250  SaveName=ScopeData22
      Scope2 settings: TimeRange=1.202697773920718e-023  YMin=0  YMax=250  SaveName=ScopeData28
      Scope4 settings: TimeRange=1.202697773920718e-023  YMin=0  YMax=250  SaveName=ScopeData30
      Scope6 settings: TimeRange=1.202697773920718e-023  YMin=0  YMax=250  SaveName=ScopeData21
  Transfer Fcn2 : TransferFcn  Numerator=[1 0]  Denominator=[0.05 1]
  Transfer Fcn3 : TransferFcn  Numerator=[1 0]  Denominator=[0.01 1]
  Transfer Fcn4 : TransferFcn  Numerator=[1 0]  Denominator=[0.01 1]
  U4 : Outport
  wires:
  angles/1 -> Bus Selector/1
  psid/1 -> Add/1, Transfer Fcn2/1
  Transfer Fcn2/1 -> Mux/2, Transfer Fcn3/1  "psiddot"
  Bus Selector/1 -> Add/2, Transfer Fcn4/1  "<psi>"
  Add/1 -> Mux/1, Integrator/1, Mux1/5, Scope6/1  "e5"
  Integrator/1 -> Mux/3, Mux1/4, Scope1/1  "X3"
  Add1/1 -> Mux1/6, Scope2/1  "e6"
  Fcn/1 -> Add1/1  "wxd"
  Mux/1 -> Fcn/1
  Mux1/1 -> Fcn1/1
  Transfer Fcn3/1 -> Mux1/3  "psiddotdot"
  Fcn1/1 -> U4/1, Scope4/1
  Transfer Fcn4/1 -> Add1/2
  omgr/1 -> Mux1/7
  Bus Selector/2 -> Mux1/1  "<phidot>"
  Bus Selector/3 -> Mux1/2  "<thetadot>"

== system IB_BIEN_y_TG_BIEN/QUADCOPTER/Inicial_conditions ==
  note: positions and linear velocities
  note: angles and angular velocities
  note: yaw
  note: pitch
  note: roll
  Bus Creator : BusCreator  Inputs=12
  phi [rad] : Constant  Value=phi0
  phidot [rad/s] : Constant  Value=phi0dot
  psi [rad] : Constant  Value=psi0
  psidot [rad/s] : Constant  Value=psi0dot
  theta [rad] : Constant  Value=theta0
  thetadot [rad/s] : Constant  Value=theta0dot
  x [m] : Constant  Value=x0
  xdot [m/s] : Constant  Value=x0dot
  y [m] : Constant  Value=y0
  ydot [m/s] : Constant  Value=y0dot
  z [m] : Constant  Value=z0
  zdot [m/s] : Constant  Value=z0dot
  Out1 : Outport
  wires:
  x [m]/1 -> Bus Creator/1  "x0"
  xdot [m/s]/1 -> Bus Creator/2  "x0dot"
  y [m]/1 -> Bus Creator/3  "y0"
  ydot [m/s]/1 -> Bus Creator/4  "y0dot"
  z [m]/1 -> Bus Creator/5  "z0"
  zdot [m/s]/1 -> Bus Creator/6  "z0dot"
  phi [rad]/1 -> Bus Creator/7  "phi0"
  phidot [rad/s]/1 -> Bus Creator/8  "phi0dot"
  theta [rad]/1 -> Bus Creator/9  "theta0"
  thetadot [rad/s]/1 -> Bus Creator/10  "theta0dot"
  psi [rad]/1 -> Bus Creator/11  "psi0"
  psidot [rad/s]/1 -> Bus Creator/12  "psi0dot"
  Bus Creator/1 -> Out1/1

== system IB_BIEN_y_TG_BIEN/QUADCOPTER/System_data ==
  Bus Creator : BusCreator  Inputs=8
  Drag Factor : Constant  Value=d
  InertiaX : Constant  Value=Ixx
  InertiaY : Constant  Value=Iyy
  InertiaZ : Constant  Value=Izz
  Length : Constant  Value=l
  Quadrotor Mass : Constant  Value=m
  Rotor Inertia : Constant  Value=Jr
  Thrust Factor : Constant  Value=b
  Out1 : Outport
  wires:
  Quadrotor Mass/1 -> Bus Creator/1  "m"
  InertiaX/1 -> Bus Creator/2  "Ixx"
  InertiaY/1 -> Bus Creator/3  "Iyy"
  InertiaZ/1 -> Bus Creator/4  "Izz"
  Thrust Factor/1 -> Bus Creator/5  "b"
  Drag Factor/1 -> Bus Creator/6  "d"
  Rotor Inertia/1 -> Bus Creator/7  "Jr"
  Length/1 -> Bus Creator/8  "l"
  Bus Creator/1 -> Out1/1

== system IB_BIEN_y_TG_BIEN/QUADCOPTER/phiddot ==
  In1 : Inport
  Bus Selector : BusSelector  OutputSignals=States.thetadot,States.psidot,omg.omg1,omg.omg2,omg.omg3,omg.omg4,data.Ixx,data.Iyy,data.Izz,data.b,data.d,data.Jr,data.l
  Fcn : Fcn  Expr=(u(1)*u(2)*u(6)/u(5))+(u(9)*u(1)*u(3)/u(5))+(u(7)*u(10)*u(4)/u(5))
  Fcn1 : Fcn  Expr=u(1)+u(3)-u(2)-u(4)
  Fcn2 : Fcn  Expr=-u(1)^2+u(2)^2
  Mux : Mux
  Mux1 : Mux  Inputs=2
  Mux2 : Mux  Inputs=10
  Subtract : Sum  Inputs=+-
  phiddot : Outport
  wires:
  In1/1 -> Bus Selector/1
  Fcn/1 -> phiddot/1
  Mux/1 -> Fcn1/1
  Mux1/1 -> Fcn2/1
  Bus Selector/3 -> Mux/1  "<omg1>"
  Bus Selector/5 -> Mux/3  "<omg3>"
  Bus Selector/6 -> Mux/4, Mux1/2  "<omg4>"
  Bus Selector/8 -> Subtract/1  "<Iyy>"
  Bus Selector/9 -> Subtract/2  "<Izz>"
  Subtract/1 -> Mux2/6
  Mux2/1 -> Fcn/1
  Fcn1/1 -> Mux2/3
  Fcn2/1 -> Mux2/4
  Bus Selector/7 -> Mux2/5  "<Ixx>"
  Bus Selector/10 -> Mux2/7  "<b>"
  Bus Selector/11 -> Mux2/8  "<d>"
  Bus Selector/12 -> Mux2/9  "<Jr>"
  Bus Selector/13 -> Mux2/10  "<l>"
  Bus Selector/4 -> Mux/2, Mux1/1  "<omg2>"
  Bus Selector/1 -> Mux2/1  "<thetadot>"
  Bus Selector/2 -> Mux2/2  "<psidot>"

== system IB_BIEN_y_TG_BIEN/QUADCOPTER/psiddot ==
  In2 : Inport
  Bus Selector : BusSelector  OutputSignals=States.phidot,States.thetadot,omg.omg1,omg.omg2,omg.omg3,omg.omg4,data.Izz,data.Ixx,data.Iyy,data.b,data.d,data.Jr
  Fcn : Fcn  Expr=(u(6)*l*u(3)/u(4))+(u(5)*u(1)*u(2)/u(4))
  Fcn1 : Fcn  Expr=-u(1)^2+u(2)^2-u(3)^2+u(4)^2
  Mux : Mux
  Mux2 : Mux  Inputs=6
  Subtract : Sum  Inputs=+-
  Terminator : Terminator
  Terminator1 : Terminator
  psiddot : Outport
  wires:
  In2/1 -> Bus Selector/1
  Fcn/1 -> psiddot/1
  Mux/1 -> Fcn1/1
  Bus Selector/3 -> Mux/1  "<omg1>"
  Bus Selector/4 -> Mux/2  "<omg2>"
  Bus Selector/5 -> Mux/3  "<omg3>"
  Bus Selector/6 -> Mux/4  "<omg4>"
  Mux2/1 -> Fcn/1
  Bus Selector/1 -> Mux2/1  "<phidot>"
  Fcn1/1 -> Mux2/3
  Bus Selector/2 -> Mux2/2  "<thetadot>"
  Bus Selector/8 -> Subtract/1  "<Ixx>"
  Bus Selector/9 -> Subtract/2  "<Iyy>"
  Bus Selector/10 -> Terminator/1  "<b>"
  Bus Selector/12 -> Terminator1/1  "<Jr>"
  Bus Selector/7 -> Mux2/4  "<Izz>"
  Subtract/1 -> Mux2/5
  Bus Selector/11 -> Mux2/6  "<d>"

== system IB_BIEN_y_TG_BIEN/QUADCOPTER/thetaddot ==
  In2 : Inport
  Bus Selector : BusSelector  OutputSignals=States.phidot,States.psidot,omg.omg1,omg.omg2,omg.omg3,omg.omg4,data.Iyy,data.Izz,data.Ixx,data.b,data.d,data.Jr,data.l
  Fcn : Fcn  Expr=(u(9)*u(1)*u(3)/u(5))+(u(6)*u(1)*u(2)/u(5))+(u(7)*u(10)*u(4)/u(5))
  Fcn1 : Fcn  Expr=-u(1)-u(3)+u(2)+u(4)
  Fcn2 : Fcn  Expr=u(1)^2-u(2)^2
  Mux : Mux
  Mux1 : Mux  Inputs=2
  Mux2 : Mux  Inputs=10
  Subtract : Sum  Inputs=+-
  thetaddot : Outport
  wires:
  In2/1 -> Bus Selector/1
  Fcn/1 -> thetaddot/1
  Mux/1 -> Fcn1/1
  Mux1/1 -> Fcn2/1
  Bus Selector/3 -> Mux/1, Mux1/2  "<omg1>"
  Bus Selector/4 -> Mux/2  "<omg2>"
  Bus Selector/5 -> Mux/3, Mux1/1  "<omg3>"
  Bus Selector/6 -> Mux/4  "<omg4>"
  Bus Selector/7 -> Mux2/5  "<Iyy>"
  Bus Selector/8 -> Subtract/1  "<Izz>"
  Mux2/1 -> Fcn/1
  Bus Selector/1 -> Mux2/1  "<phidot>"
  Fcn1/1 -> Mux2/3
  Fcn2/1 -> Mux2/4
  Bus Selector/10 -> Mux2/7  "<b>"
  Bus Selector/11 -> Mux2/8  "<d>"
  Bus Selector/12 -> Mux2/9  "<Jr>"
  Bus Selector/9 -> Subtract/2  "<Ixx>"
  Subtract/1 -> Mux2/6
  Bus Selector/13 -> Mux2/10  "<l>"
  Bus Selector/2 -> Mux2/2  "<psidot>"

== system IB_BIEN_y_TG_BIEN/QUADCOPTER/xddot ==
  In1 : Inport
  Bus Selector : BusSelector  OutputSignals=data.m,data.b,omg.omg1,omg.omg2,omg.omg3,omg.omg4,States.phi,States.theta,States.psi
  Fcn : Fcn  Expr=u(2)*(u(3)^2+u(4)^2+u(5)^2+u(6)^2)/u(1)
  Fcn1 : Fcn  Expr=u(1)*(cos(u(2))*sin(u(3))*cos(u(4))+sin(u(2))*sin(u(4)))
  Mux : Mux  Inputs=6
  Mux3 : Mux
  xdotdot : Outport
  wires:
  In1/1 -> Bus Selector/1
  Bus Selector/1 -> Mux/1  "<m>"
  Bus Selector/2 -> Mux/2  "<b>"
  Bus Selector/3 -> Mux/3  "<omg1>"
  Bus Selector/4 -> Mux/4  "<omg2>"
  Bus Selector/5 -> Mux/5  "<omg3>"
  Bus Selector/6 -> Mux/6  "<omg4>"
  Mux/1 -> Fcn/1
  Fcn1/1 -> xdotdot/1
  Mux3/1 -> Fcn1/1
  Fcn/1 -> Mux3/1
  Bus Selector/7 -> Mux3/2  "<phi>"
  Bus Selector/8 -> Mux3/3  "<theta>"
  Bus Selector/9 -> Mux3/4  "<psi>"

== system IB_BIEN_y_TG_BIEN/QUADCOPTER/yddot ==
  In1 : Inport
  Bus Selector : BusSelector  OutputSignals=data.m,data.b,omg.omg1,omg.omg2,omg.omg3,omg.omg4,States.phi,States.theta,States.psi
  Fcn : Fcn  Expr=u(2)*(u(3)^2+u(4)^2+u(5)^2+u(6)^2)/u(1)
  Fcn1 : Fcn  Expr=u(1)*(cos(u(2))*sin(u(3))*sin(u(4))-sin(u(2))*cos(u(4)))
  Mux : Mux  Inputs=6
  Mux3 : Mux
  ydotdot : Outport
  wires:
  In1/1 -> Bus Selector/1
  Bus Selector/1 -> Mux/1  "<m>"
  Bus Selector/2 -> Mux/2  "<b>"
  Bus Selector/3 -> Mux/3  "<omg1>"
  Bus Selector/4 -> Mux/4  "<omg2>"
  Bus Selector/5 -> Mux/5  "<omg3>"
  Bus Selector/6 -> Mux/6  "<omg4>"
  Mux/1 -> Fcn/1
  Fcn1/1 -> ydotdot/1
  Mux3/1 -> Fcn1/1
  Fcn/1 -> Mux3/1
  Bus Selector/7 -> Mux3/2  "<phi>"
  Bus Selector/8 -> Mux3/3  "<theta>"
  Bus Selector/9 -> Mux3/4  "<psi>"

== system IB_BIEN_y_TG_BIEN/QUADCOPTER/zddot ==
  In1 : Inport
  Bus Selector : BusSelector  OutputSignals=data.m,data.b,omg.omg1,omg.omg2,omg.omg3,omg.omg4,States.phi,States.theta
  Fcn : Fcn  Expr=u(2)*(u(3)^2+u(4)^2+u(5)^2+u(6)^2)/u(1)
  Fcn1 : Fcn  Expr=(u(2)*cos(u(3))*cos(u(4)))-u(1)
  Mux : Mux  Inputs=6
  Mux3 : Mux
  gravity : Constant  Value=9.81
  zdotdot : Outport
  wires:
  In1/1 -> Bus Selector/1
  Bus Selector/1 -> Mux/1  "<m>"
  Bus Selector/2 -> Mux/2  "<b>"
  Bus Selector/3 -> Mux/3  "<omg1>"
  Bus Selector/4 -> Mux/4  "<omg2>"
  Bus Selector/5 -> Mux/5  "<omg3>"
  Bus Selector/6 -> Mux/6  "<omg4>"
  Mux/1 -> Fcn/1
  Fcn1/1 -> zdotdot/1
  Mux3/1 -> Fcn1/1
  gravity/1 -> Mux3/1
  Fcn/1 -> Mux3/2
  Bus Selector/7 -> Mux3/3  "<phi>"
  Bus Selector/8 -> Mux3/4  "<theta>"

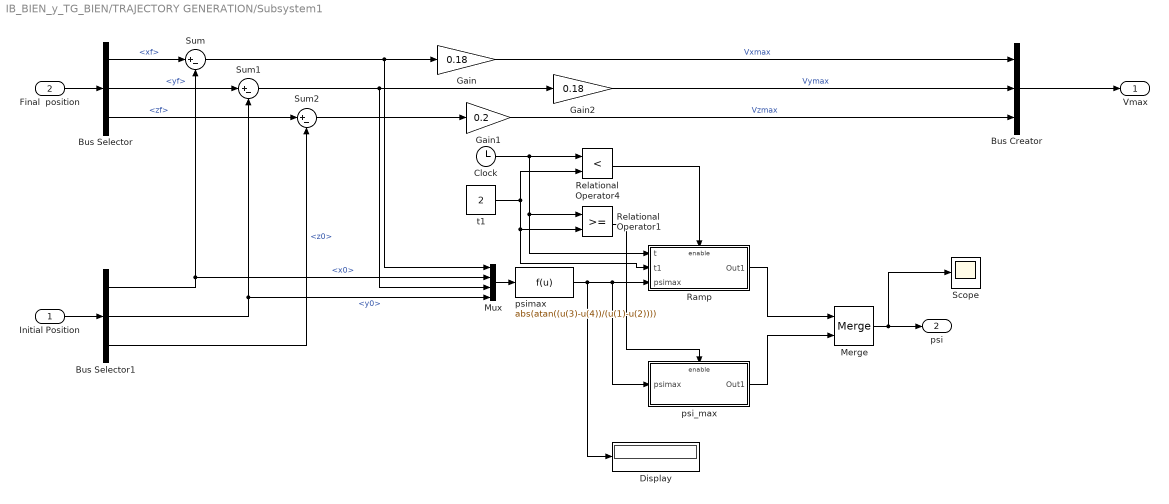
== system IB_BIEN_y_TG_BIEN/TRAJECTORY GENERATION/Subsystem1 ==
  Initial Position : Inport
  Final  position : Inport  Port=2
  Bus Creator : BusCreator  Inputs=3
  Bus Selector : BusSelector  OutputSignals=xf,yf,zf
  Bus Selector1 : BusSelector  OutputSignals=x0,y0,z0
  Clock : Clock
  Display : Display
  Gain : Gain  Gain=0.18
  Gain1 : Gain  Gain=0.2
  Gain2 : Gain  Gain=0.18
  Merge : Merge
  Mux : Mux
  Ramp : Subsystem  TreatAsAtomicUnit=on
  Relational Operator1 : RelationalOperator  OutDataTypeStr=boolean
  Relational Operator4 : RelationalOperator  Operator=<  OutDataTypeStr=boolean
  Scope : Scope
      settings: SaveName=ScopeData10
  Sum : Sum  Inputs=|+-
  Sum1 : Sum  Inputs=|+-
  Sum2 : Sum  Inputs=|+-
  psi_max : Subsystem  TreatAsAtomicUnit=on
  psimax : Fcn  Expr=abs(atan((u(3)-u(4))/(u(1)-u(2))))
  t1 : Constant  Value=2
  Vmax : Outport
  psi : Outport  Port=2
  wires:
  Bus Creator/1 -> Vmax/1
  Final  position/1 -> Bus Selector/1
  Initial Position/1 -> Bus Selector1/1
  Bus Selector/2 -> Sum1/1  "<yf>"
  Bus Selector1/2 -> Sum1/2, Mux/4  "<y0>"
  Bus Selector/1 -> Sum/1  "<xf>"
  Bus Selector1/1 -> Sum/2, Mux/2  "<x0>"
  Bus Selector/3 -> Sum2/1  "<zf>"
  Bus Selector1/3 -> Sum2/2  "<z0>"
  Gain/1 -> Bus Creator/1  "Vxmax"
  Gain2/1 -> Bus Creator/2  "Vymax"
  Gain1/1 -> Bus Creator/3  "Vzmax"
  Sum/1 -> Gain/1, Mux/1
  Sum2/1 -> Gain1/1
  Sum1/1 -> Gain2/1, Mux/3
  Clock/1 -> Relational Operator4/1, Relational Operator1/1, Ramp/1(t)
  Merge/1 -> psi/1, Scope/1
  t1/1 -> Relational Operator4/2, Relational Operator1/2, Ramp/2(t1)
  Mux/1 -> psimax/1
  Ramp/1(Out1) -> Merge/1
  psi_max/1(Out1) -> Merge/2
  Relational Operator4/1 -> Ramp/Enable
  Relational Operator1/1 -> psi_max/Enable
  psimax/1 -> Ramp/3(psimax), psi_max/1(psimax), Display/1

== system IB_BIEN_y_TG_BIEN/TRAJECTORY GENERATION/Subsystem5 ==
  Positions : Inport
  Initial_position : Inport  Port=2
  Bus Creator : BusCreator  Inputs=3
  Bus Selector : BusSelector  OutputSignals=x,y,z
  Bus Selector1 : BusSelector  OutputSignals=x0,y0,z0
  Clock : Clock
  Constant : Constant  Value=0
  Display{,1..4} (5 alike) : Display
  Subsystem : Subsystem
  Subsystem1 : Subsystem
  Subsystem2 : Subsystem
  Position : Outport
  wires:
  Bus Creator/1 -> Position/1
  Positions/1 -> Bus Selector/1
  Initial_position/1 -> Bus Selector1/1
  Bus Selector/1 -> Display1/1  "<x>"
  Bus Selector1/1 -> Subsystem/3(x_ent0)  "<x0>"
  Subsystem/1(x0) -> Bus Creator/1, Display/1  "x"
  Clock/1 -> Subsystem/1(t), Subsystem1/1(t), Subsystem2/1(t)
  Constant/1 -> Subsystem/2(0), Subsystem1/2(In2), Subsystem2/2(In2)
  Subsystem1/1(y0) -> Bus Creator/2  "y"
  Subsystem2/1(z0) -> Bus Creator/3, Display2/1  "z"
  Bus Selector/2 -> Display3/1  "<y>"
  Bus Selector/3 -> Display4/1  "<z>"
  Bus Selector1/2 -> Subsystem1/3(y_ent0)  "<y0>"
  Bus Selector1/3 -> Subsystem2/3(z_ent0)  "<z0>"

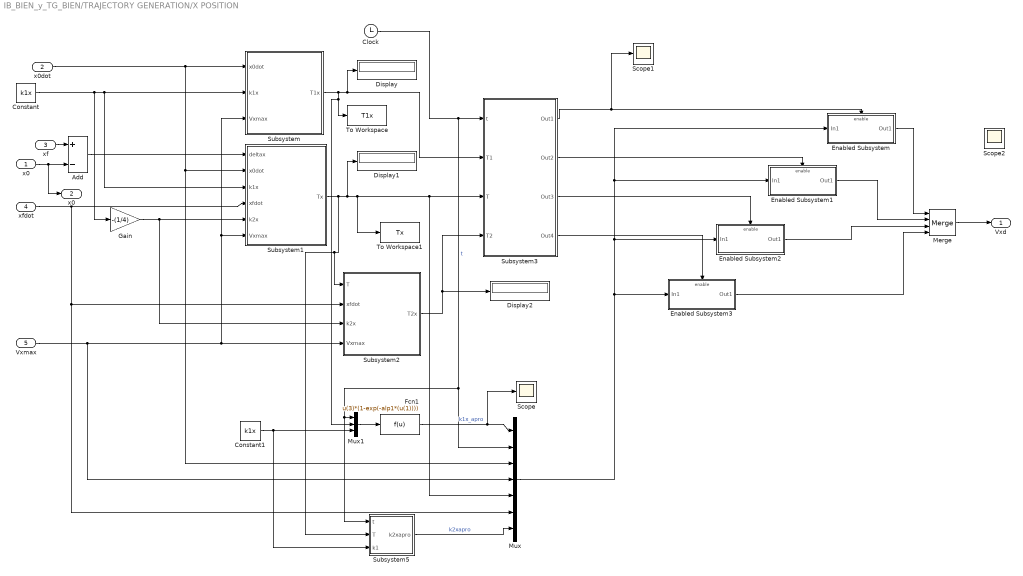
== system IB_BIEN_y_TG_BIEN/TRAJECTORY GENERATION/X POSITION ==
  x0 : Inport
  x0dot : Inport  Port=2
  xf : Inport  Port=3
  xfdot : Inport  Port=4
  Vxmax : Inport  Port=5
  Add : Sum  Inputs=+-
  Clock : Clock
  Constant : Constant  Value=k1x
  Constant1 : Constant  Value=k1x
  Display : Display
  Display1 : Display
  Display2 : Display
  Enabled Subsystem : Subsystem  TreatAsAtomicUnit=on
  Enabled Subsystem1 : Subsystem  TreatAsAtomicUnit=on
  Enabled Subsystem2 : Subsystem  TreatAsAtomicUnit=on
  Enabled Subsystem3 : Subsystem  TreatAsAtomicUnit=on
  Fcn1 : Fcn  Expr=u(3)*(1-exp(-alp1*(u(1))))
  Gain : Gain  Gain=-(1/4)
  Merge : Merge  Inputs=4
  Mux : Mux  Inputs=7
  Mux1 : Mux  Inputs=3
  Scope : Scope
      settings: SaveName=ScopeData3
  Scope1 : Scope
      settings: SaveName=ScopeData4
  Scope2 : Scope
      settings: SaveName=ScopeData5
  Subsystem : Subsystem
  Subsystem1 : Subsystem
  Subsystem2 : Subsystem
  Subsystem3 : Subsystem
  Subsystem5 : Subsystem
  To Workspace : ToWorkspace  VariableName=T1x  SampleTime=-1
  To Workspace1 : ToWorkspace  VariableName=Tx  SampleTime=-1
  Vxd : Outport
  "x0 " : Outport  Port=2
  wires:
  x0dot/1 -> Subsystem/1(x0dot), Subsystem1/2(x0dot), Mux/3
  xfdot/1 -> Subsystem1/4(xfdot), Subsystem2/2(xfdot), Mux/6
  Subsystem1/1(Tx) -> Display1/1, Subsystem3/3(T), Mux/5, To Workspace1/1, Subsystem2/1(T), Subsystem5/2(T)
  Clock/1 -> Subsystem3/1(t), Mux/2, Mux1/1, Subsystem5/1(t)  "t"
  Subsystem3/1(Out1) -> Enabled Subsystem/Enable, Scope1/1
  Subsystem3/2(Out2) -> Enabled Subsystem1/Enable
  Subsystem3/4(Out4) -> Enabled Subsystem3/Enable
  Subsystem3/3(Out3) -> Enabled Subsystem2/Enable
  Subsystem/1(T1x) -> Subsystem3/2(T1), Display/1, To Workspace/1, Mux1/2
  Subsystem2/1(T2x) -> Subsystem3/4(T2), Display2/1
  Mux/1 -> Enabled Subsystem3/1(In1), Enabled Subsystem2/1(In1), Enabled Subsystem1/1(In1), Enabled Subsystem/1(In1)
  Enabled Subsystem/1(Out1) -> Merge/1
  Enabled Subsystem1/1(Out1) -> Merge/2
  Enabled Subsystem2/1(Out1) -> Merge/3
  Enabled Subsystem3/1(Out1) -> Merge/4
  Merge/1 -> Vxd/1
  Vxmax/1 -> Subsystem/3(Vxmax), Subsystem1/6(Vxmax), Subsystem2/4(Vxmax), Mux/4
  Constant/1 -> Subsystem/2(k1x), Subsystem1/3(k1x), Gain/1
  Gain/1 -> Subsystem1/5(k2x), Subsystem2/3(k2x)
  Mux1/1 -> Fcn1/1
  Fcn1/1 -> Mux/1, Scope/1  "k1x_apro"
  Constant1/1 -> Mux1/3, Subsystem5/3(k1)
  Subsystem5/1(k2xapro) -> Mux/7  "k2xapro"
  xf/1 -> Add/1
  x0/1 -> Add/2, "x0 "/1
  Add/1 -> Subsystem1/1(deltax)

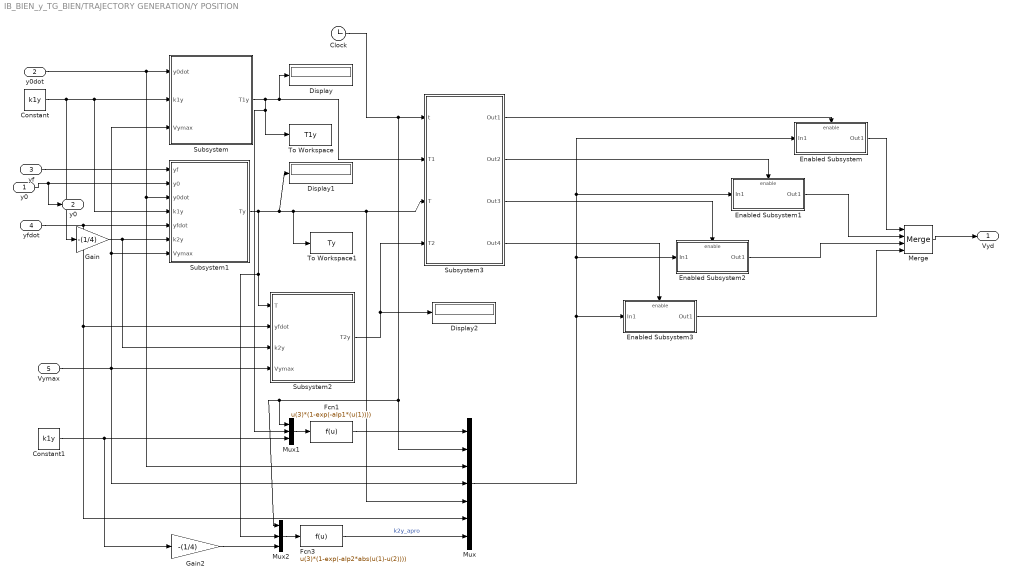
== system IB_BIEN_y_TG_BIEN/TRAJECTORY GENERATION/Y POSITION ==
  y0 : Inport
  y0dot : Inport  Port=2
  yf : Inport  Port=3
  yfdot : Inport  Port=4
  Vymax : Inport  Port=5
  Clock : Clock
  Constant : Constant  Value=k1y
  Constant1 : Constant  Value=k1y
  Display : Display
  Display1 : Display
  Display2 : Display
  Enabled Subsystem : Subsystem  TreatAsAtomicUnit=on
  Enabled Subsystem1 : Subsystem  TreatAsAtomicUnit=on
  Enabled Subsystem2 : Subsystem  TreatAsAtomicUnit=on
  Enabled Subsystem3 : Subsystem  TreatAsAtomicUnit=on
  Fcn1 : Fcn  Expr=u(3)*(1-exp(-alp1*(u(1))))
  Fcn3 : Fcn  Expr=u(3)*(1-exp(-alp2*abs(u(1)-u(2))))
  Gain : Gain  Gain=-(1/4)
  Gain2 : Gain  Gain=-(1/4)
  Merge : Merge  Inputs=4
  Mux : Mux  Inputs=7
  Mux1 : Mux  Inputs=3
  Mux2 : Mux  Inputs=3
  Subsystem : Subsystem
  Subsystem1 : Subsystem
  Subsystem2 : Subsystem
  Subsystem3 : Subsystem
  To Workspace : ToWorkspace  VariableName=T1y  SampleTime=-1
  To Workspace1 : ToWorkspace  VariableName=Ty  SampleTime=-1
  Vyd : Outport
  "y0  " : Outport  Port=2
  wires:
  y0/1 -> Subsystem1/2(y0), "y0  "/1
  yf/1 -> Subsystem1/1(yf)
  y0dot/1 -> Subsystem/1(y0dot), Subsystem1/3(y0dot), Mux/3
  yfdot/1 -> Subsystem1/5(yfdot), Subsystem2/2(yfdot), Mux/6
  Subsystem1/1(Ty) -> Display1/1, Subsystem3/3(T), Mux/5, To Workspace1/1, Subsystem2/1(T), Mux2/2
  Clock/1 -> Subsystem3/1(t), Mux/2, Mux1/1, Mux2/1
  Subsystem3/1(Out1) -> Enabled Subsystem/Enable
  Subsystem3/2(Out2) -> Enabled Subsystem1/Enable
  Subsystem3/4(Out4) -> Enabled Subsystem3/Enable
  Subsystem3/3(Out3) -> Enabled Subsystem2/Enable
  Subsystem/1(T1y) -> Subsystem3/2(T1), Display/1, To Workspace/1, Mux1/2
  Subsystem2/1(T2y) -> Subsystem3/4(T2), Display2/1
  Vymax/1 -> Subsystem1/7(Vymax), Subsystem/3(Vymax), Subsystem2/4(Vymax), Mux/4
  Mux/1 -> Enabled Subsystem3/1(In1), Enabled Subsystem2/1(In1), Enabled Subsystem1/1(In1), Enabled Subsystem/1(In1)
  Enabled Subsystem/1(Out1) -> Merge/1
  Enabled Subsystem1/1(Out1) -> Merge/2
  Enabled Subsystem2/1(Out1) -> Merge/3
  Enabled Subsystem3/1(Out1) -> Merge/4
  Merge/1 -> Vyd/1
  Constant/1 -> Subsystem/2(k1y), Subsystem1/4(k1y), Gain/1
  Gain/1 -> Subsystem1/6(k2y), Subsystem2/3(k2y)
  Mux1/1 -> Fcn1/1
  Fcn1/1 -> Mux/1
  Constant1/1 -> Mux1/3, Gain2/1
  Mux2/1 -> Fcn3/1
  Gain2/1 -> Mux2/3
  Fcn3/1 -> Mux/7  "k2y_apro"

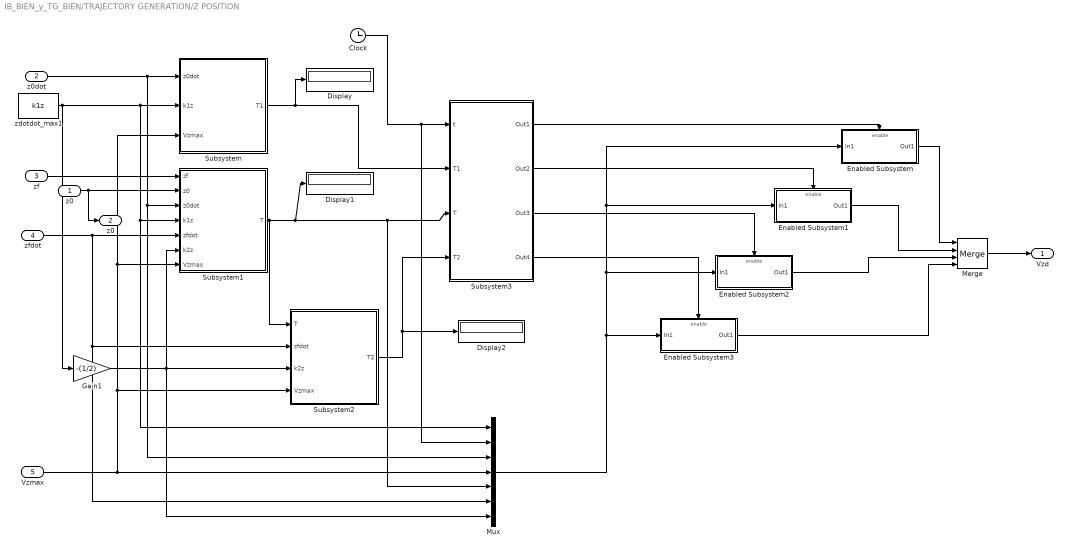
== system IB_BIEN_y_TG_BIEN/TRAJECTORY GENERATION/Z POSITION ==
  z0 : Inport
  z0dot : Inport  Port=2
  zf : Inport  Port=3
  zfdot : Inport  Port=4
  Vzmax : Inport  Port=5
  Clock : Clock
  Display : Display
  Display1 : Display
  Display2 : Display
  Enabled Subsystem : Subsystem  TreatAsAtomicUnit=on
  Enabled Subsystem1 : Subsystem  TreatAsAtomicUnit=on
  Enabled Subsystem2 : Subsystem  TreatAsAtomicUnit=on
  Enabled Subsystem3 : Subsystem  TreatAsAtomicUnit=on
  Gain1 : Gain  Gain=-(1/2)
  Merge : Merge  Inputs=4
  Mux : Mux  Inputs=7
  Subsystem : Subsystem
  Subsystem1 : Subsystem
  Subsystem2 : Subsystem
  Subsystem3 : Subsystem
  zdotdot_max1 : Constant  Value=k1z
  Vzd : Outport
  "z0 " : Outport  Port=2
  wires:
  z0/1 -> Subsystem1/2(z0), "z0 "/1
  zf/1 -> Subsystem1/1(zf)
  z0dot/1 -> Subsystem/1(z0dot), Subsystem1/3(z0dot), Mux/3
  zdotdot_max1/1 -> Subsystem/2(k1z), Subsystem1/4(k1z), Mux/1, Gain1/1
  zfdot/1 -> Subsystem1/5(zfdot), Subsystem2/2(zfdot), Mux/6
  Subsystem1/1(T) -> Subsystem2/1(T), Subsystem3/3(T), Mux/5, Display1/1
  Clock/1 -> Subsystem3/1(t), Mux/2
  Subsystem3/1(Out1) -> Enabled Subsystem/Enable
  Subsystem3/2(Out2) -> Enabled Subsystem1/Enable
  Subsystem3/4(Out4) -> Enabled Subsystem3/Enable
  Subsystem3/3(Out3) -> Enabled Subsystem2/Enable
  Subsystem/1(T1) -> Subsystem3/2(T1), Display/1
  Subsystem2/1(T2) -> Subsystem3/4(T2), Display2/1
  Vzmax/1 -> Mux/4, Subsystem2/4(Vzmax), Subsystem/3(Vzmax), Subsystem1/7(Vzmax)
  Mux/1 -> Enabled Subsystem3/1(In1), Enabled Subsystem2/1(In1), Enabled Subsystem1/1(In1), Enabled Subsystem/1(In1)
  Enabled Subsystem/1(Out1) -> Merge/1
  Enabled Subsystem1/1(Out1) -> Merge/2
  Enabled Subsystem2/1(Out1) -> Merge/3
  Enabled Subsystem3/1(Out1) -> Merge/4
  Merge/1 -> Vzd/1
  Gain1/1 -> Subsystem2/3(k2z), Subsystem1/6(k2z), Mux/7

== system IB_BIEN_y_TG_BIEN/X POSITION CONTROL IB/Position Control ==
  In2 : Inport
  Trigger : TriggerPort  PortDimensions=1
  thetad : Outport
  wires:
  In2/1 -> thetad/1

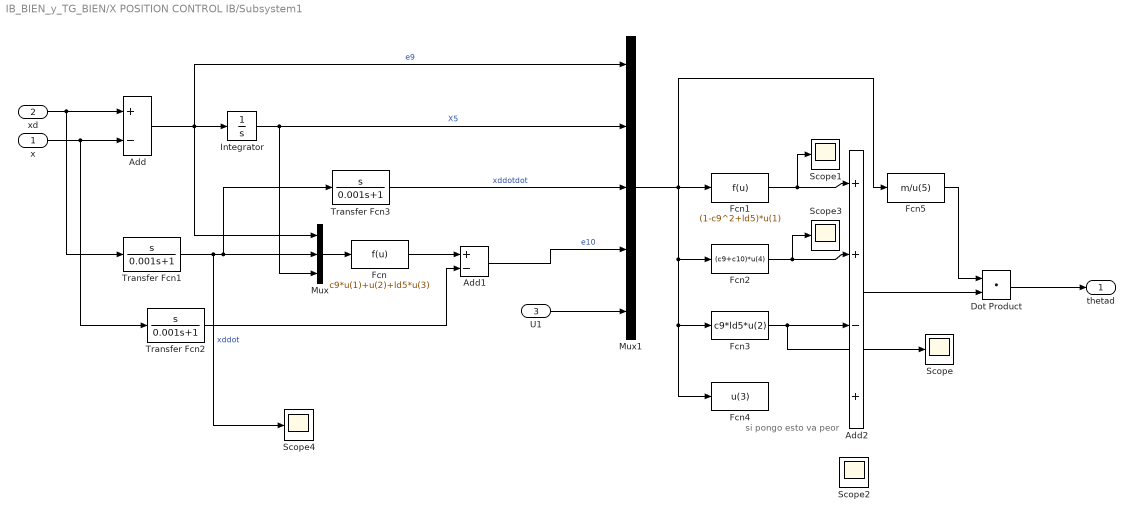
== system IB_BIEN_y_TG_BIEN/X POSITION CONTROL IB/Subsystem1 ==
  note: si pongo esto va peor
  x : Inport
  xd : Inport  Port=2
  U1 : Inport  Port=3
  Add : Sum  Inputs=+-
  Add1 : Sum  Inputs=+-
  Add2 : Sum  Inputs=++-+
  Dot Product : DotProduct  InputSameDT=on  OutDataTypeStr=Inherit: Inherit via internal rule
  Fcn : Fcn  Expr=c9*u(1)+u(2)+ld5*u(3)
  Fcn1 : Fcn  Expr=(1-c9^2+ld5)*u(1)
  Fcn2 : Fcn  Expr=(c9+c10)*u(4)
  Fcn3 : Fcn  Expr=c9*ld5*u(2)
  Fcn4 : Fcn  Expr=u(3)
  Fcn5 : Fcn  Expr=m/u(5)
  Integrator : Integrator
  Mux : Mux  Inputs=3
  Mux1 : Mux  Inputs=5
  Scope{,1..4} (5 alike) : Scope
      Scope settings: SaveName=ScopeData17
      Scope1 settings: SaveName=ScopeData25
      Scope2 settings: SaveName=ScopeData26
      Scope3 settings: SaveName=ScopeData27
      Scope4 settings: SaveName=ScopeData2
  Transfer Fcn1 : TransferFcn  Numerator=[1 0]  Denominator=[0.001 1]
  Transfer Fcn2 : TransferFcn  Numerator=[1 0]  Denominator=[0.001 1]
  Transfer Fcn3 : TransferFcn  Numerator=[1 0]  Denominator=[0.001 1]
  thetad : Outport
  wires:
  xd/1 -> Add/1, Transfer Fcn1/1
  x/1 -> Add/2, Transfer Fcn2/1
  Add/1 -> Integrator/1, Mux/1, Mux1/1  "e9"
  Integrator/1 -> Mux/3, Mux1/2  "X5"
  Transfer Fcn1/1 -> Mux/2, Transfer Fcn3/1, Scope4/1  "xddot"
  Mux/1 -> Fcn/1
  Fcn/1 -> Add1/1
  Transfer Fcn2/1 -> Add1/2
  U1/1 -> Mux1/5
  Add1/1 -> Mux1/4  "e10"
  Transfer Fcn3/1 -> Mux1/3  "xddotdot"
  Mux1/1 -> Fcn1/1, Fcn2/1, Fcn3/1, Fcn4/1, Fcn5/1
  Fcn1/1 -> Add2/1, Scope1/1
  Fcn2/1 -> Add2/2, Scope3/1
  Fcn3/1 -> Add2/3, Scope/1
  Add2/1 -> Dot Product/2
  Fcn5/1 -> Dot Product/1
  Dot Product/1 -> thetad/1

== system IB_BIEN_y_TG_BIEN/Y POSITION CONTROL IB/Position Control ==
  In2 : Inport
  Trigger : TriggerPort  PortDimensions=1
  phid : Outport
  wires:
  In2/1 -> phid/1

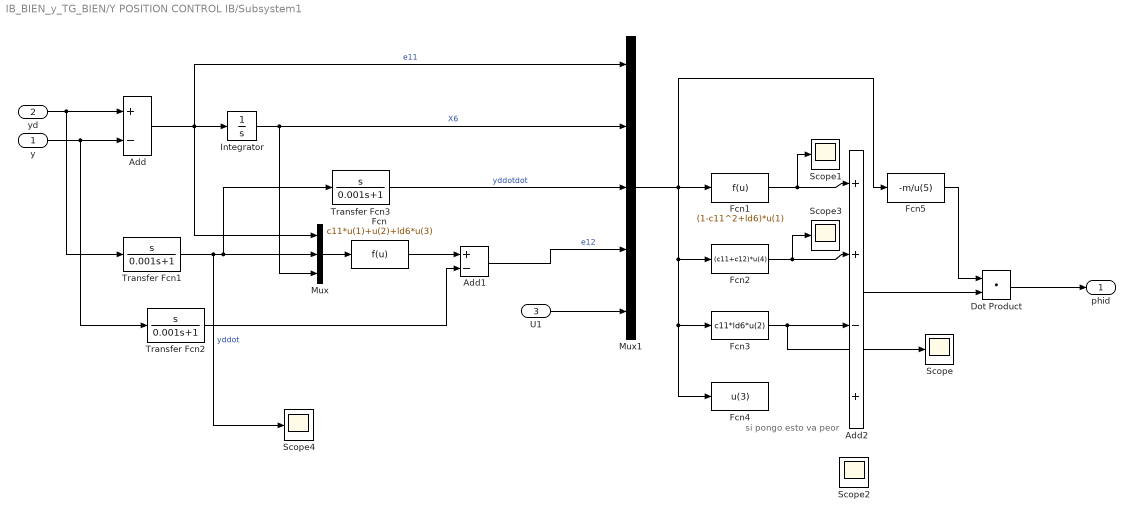
== system IB_BIEN_y_TG_BIEN/Y POSITION CONTROL IB/Subsystem1 ==
  note: si pongo esto va peor
  y : Inport
  yd : Inport  Port=2
  U1 : Inport  Port=3
  Add : Sum  Inputs=+-
  Add1 : Sum  Inputs=+-
  Add2 : Sum  Inputs=++-+
  Dot Product : DotProduct  InputSameDT=on  OutDataTypeStr=Inherit: Inherit via internal rule
  Fcn : Fcn  Expr=c11*u(1)+u(2)+ld6*u(3)
  Fcn1 : Fcn  Expr=(1-c11^2+ld6)*u(1)
  Fcn2 : Fcn  Expr=(c11+c12)*u(4)
  Fcn3 : Fcn  Expr=c11*ld6*u(2)
  Fcn4 : Fcn  Expr=u(3)
  Fcn5 : Fcn  Expr=-m/u(5)
  Integrator : Integrator
  Mux : Mux  Inputs=3
  Mux1 : Mux  Inputs=5
  Scope{,1..4} (5 alike) : Scope
      Scope settings: SaveName=ScopeData17
      Scope1 settings: SaveName=ScopeData25
      Scope2 settings: SaveName=ScopeData26
      Scope3 settings: SaveName=ScopeData27
      Scope4 settings: SaveName=ScopeData2
  Transfer Fcn1 : TransferFcn  Numerator=[1 0]  Denominator=[0.001 1]
  Transfer Fcn2 : TransferFcn  Numerator=[1 0]  Denominator=[0.001 1]
  Transfer Fcn3 : TransferFcn  Numerator=[1 0]  Denominator=[0.001 1]
  phid : Outport
  wires:
  yd/1 -> Add/1, Transfer Fcn1/1
  y/1 -> Add/2, Transfer Fcn2/1
  Add/1 -> Integrator/1, Mux/1, Mux1/1  "e11"
  Integrator/1 -> Mux/3, Mux1/2  "X6"
  Transfer Fcn1/1 -> Mux/2, Transfer Fcn3/1, Scope4/1  "yddot"
  Mux/1 -> Fcn/1
  Fcn/1 -> Add1/1
  Transfer Fcn2/1 -> Add1/2
  U1/1 -> Mux1/5
  Add1/1 -> Mux1/4  "e12"
  Transfer Fcn3/1 -> Mux1/3  "yddotdot"
  Mux1/1 -> Fcn1/1, Fcn2/1, Fcn3/1, Fcn4/1, Fcn5/1
  Fcn1/1 -> Add2/1, Scope1/1
  Fcn2/1 -> Add2/2, Scope3/1
  Fcn3/1 -> Add2/3, Scope/1
  Add2/1 -> Dot Product/2
  Fcn5/1 -> Dot Product/1
  Dot Product/1 -> phid/1

== system IB_BIEN_y_TG_BIEN/TRAJECTORY GENERATION/Subsystem1/Ramp ==
  t : Inport
  t1 : Inport  Port=2
  psimax : Inport  Port=3
  Enable : EnablePort
  Fcn : Fcn  Expr=(u(1)/u(3))*u(2)
  Mux : Mux  Inputs=3
  Out1 : Outport
  wires:
  Fcn/1 -> Out1/1
  Mux/1 -> Fcn/1
  psimax/1 -> Mux/1
  t/1 -> Mux/2
  t1/1 -> Mux/3

== system IB_BIEN_y_TG_BIEN/TRAJECTORY GENERATION/Subsystem1/psi_max ==
  psimax : Inport
  Enable : EnablePort
  Out1 : Outport
  wires:
  psimax/1 -> Out1/1

== system IB_BIEN_y_TG_BIEN/TRAJECTORY GENERATION/Subsystem5/Subsystem ==
  t : Inport
  0 : Inport  Port=2
  x_ent0 : Inport  Port=3
  Display2 : Display
  Enabled Subsystem : Subsystem  TreatAsAtomicUnit=on
  Enabled Subsystem1 : Subsystem  TreatAsAtomicUnit=on
  Merge : Merge
  Relational Operator : RelationalOperator  Operator===  OutDataTypeStr=boolean
  Relational Operator1 : RelationalOperator  Operator=~=  OutDataTypeStr=boolean
  Scope : Scope
  Scope1 : Scope
      settings: SaveName=ScopeData6
  x0 : Outport
  wires:
  t/1 -> Relational Operator1/1, Relational Operator/1
  0/1 -> Relational Operator/2, Relational Operator1/2, Enabled Subsystem1/1(In1)
  Relational Operator/1 -> Enabled Subsystem/Enable
  Enabled Subsystem/1(Out1) -> Merge/1
  Relational Operator1/1 -> Enabled Subsystem1/Enable, Scope/1
  Enabled Subsystem1/1(Out1) -> Merge/2
  x_ent0/1 -> Enabled Subsystem/1(In1)
  Merge/1 -> Display2/1, x0/1, Scope1/1
